simulink model "LQR_integration"  (Simulink 10.1)
settings: Solver=ode45  StartTime=0.0  StopTime=10  FixedStep=0.01  RelTol=1e-3  EnableMultiTasking=on
values from neighbouring files (symbols this model uses):
  A = [1 3 ... (first row only)    [Task_3.m]    (also in Task_5.m = [-1.460,0, 2.4276)
  B = [1 ... (first row only)    [Task_3.m]    (also in Task_5.m = [0.4182, 5.2026)
  Kr = lqr(A_aug,B_aug,Q,R)    [Task_5.m]
  r1 = r(i,1)    [Task_5.m]
  r2 = r(i,2)    [Task_5.m]
settings Model: Creator=tonia  LastModifiedBy=gkass
settings DataIOCC: LimitDataPoints=on  SignalLoggingSaveFormat=ModelDataLogs
settings OptimizationCC: ExpressionDepthLimit=2147483647
settings DebuggingCC: SolverPrmCheckMsg=warning  FcnCallInpInsideContextMsg=warning  StateNameClashWarn=warning

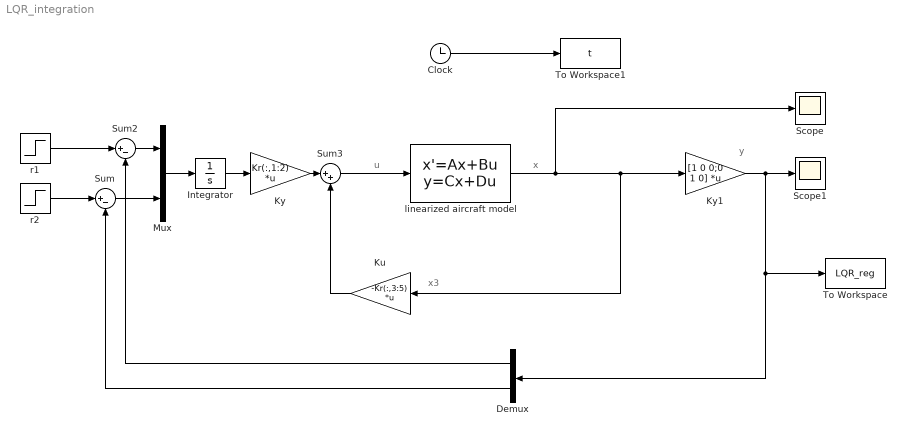
== system LQR_integration ==
  note: y
  note: x3
  note: u
  note: x
  Clock : Clock
  Demux : Demux  Outputs=2
  Integrator : Integrator
  Ku : Gain  Gain=-Kr(:,3:5)  Multiplication=Matrix(K*u)  ParamDataTypeStr=Inherit: Same as input
  Ky : Gain  Gain=Kr(:,1:2)  Multiplication=Matrix(K*u)  ParamDataTypeStr=Inherit: Same as input
  Ky1 : Gain  Gain=[1 0 0;0 1 0]  Multiplication=Matrix(K*u)  ParamDataTypeStr=Inherit: Same as input
  Mux : Mux  Inputs=2
  Scope : Scope
  Scope1 : Scope
  Sum : Sum  Inputs=|+-
  Sum2 : Sum  Inputs=|+-
  Sum3 : Sum  Inputs=|++
  To Workspace : ToWorkspace  VariableName=LQR_reg  SampleTime=-1
  To Workspace1 : ToWorkspace  VariableName=t  SampleTime=-1
  linearized aircraft model : StateSpace  A=A  B=B  C=eye(3)  D=zeros(3,2)  InitialCondition=[0 0 0]
  r1 : Step  Time=0  After=r1  SampleTime=0
  r2 : Step  Time=0  After=r2  SampleTime=1
  wires:
  linearized aircraft model/1 -> Scope/1, Ky1/1, Ku/1
  r1/1 -> Sum2/1
  r2/1 -> Sum/1
  Ku/1 -> Sum3/2
  Sum3/1 -> linearized aircraft model/1
  Demux/1 -> Sum2/2
  Demux/2 -> Sum/2
  Ky/1 -> Sum3/1
  Sum2/1 -> Mux/1
  Sum/1 -> Mux/2
  Clock/1 -> To Workspace1/1
  Ky1/1 -> Scope1/1, Demux/1, To Workspace/1
  Mux/1 -> Integrator/1
  Integrator/1 -> Ky/1
